simulink model "A2V5"  (R2021b)
settings: Solver=FixedStepAuto  StartTime=0.0  StopTime=10.0  FixedStep=1e-3  RelTol=1e-3  EnableMultiTasking=on
undefined symbols (not defined in the file): a, A0, A1, b, c, D0, D1, D10, D11, D12, D13, D2, D3, D4, D5, D6, D7, D8, D9, magnitude, PTA0, PTA1, PTA2, PTB2, PTB23, PTB3, PTB9, PTC16, PTC17, PTC2, PTC3, PTC4, PTD0, PTD1, PTD2, PTD3
libraries: frdmk64flib x23, etargetslib x21, simulink x2, dspstat3 x1, hdlsllib x1
settings Model: ExtModeTrigDuration=5  Creator=adamj  LastModifiedBy=adamj
settings OptimizationCC: EnhancedBackFolding=on  PassReuseOutputArgsAs=Individual arguments  ZeroExternalMemoryAtStartup=off  ZeroInternalMemoryAtStartup=off  MaxStackSize=64  OptimizeBlockOrder=speed  DifferentSizesBufferReuse=on  OptimizationCustomize=off  EfficientTunableParamExpr=on
settings DebuggingCC: ParameterTunabilityLossMsg=error
settings HardwareCC: ProdBitPerPointer=32  ProdBitPerSizeT=32  ProdBitPerPtrDiffT=32  ProdLargestAtomicInteger=Long  ProdLargestAtomicFloat=Double  ProdWordSize=32  ProdHWDeviceType=ARM Compatible->ARM Cortex
settings SFSimCC: MATLABDynamicMemAlloc=off
settings RTWCC: Description=Embedded Coder  SystemTargetFile=ert.tlc  HardwareBoard=NXP FRDM-K64F  TLCOptions="-aInlineSetEventsForThisBaseRateFcn=TLC_FALSE -aSuppressMultiTaskScheduler=TLC_FALSE  -aRateBasedStepFcn=0"  TemplateMakefile=ert_default_tmf  Toolchain=GNU Tools for ARM Embedded Processors
settings CodeAppCC: ForceParamTrailComments=on  IgnoreCustomStorageClasses=off  OperatorAnnotations=on  SimulinkDataObjDesc=on  SFDataObjDesc=on  InsertBlockDesc=on
settings ERTTargetCC: ExtModeTransport=4  ExtModeMexFile=sendToCommService

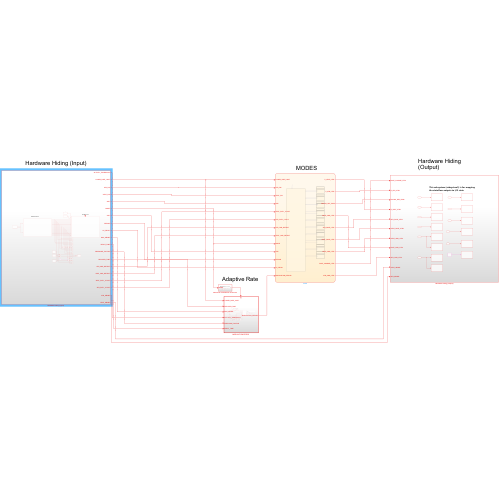
[thumbnail: Simulink's stored preview of the top-level diagram]
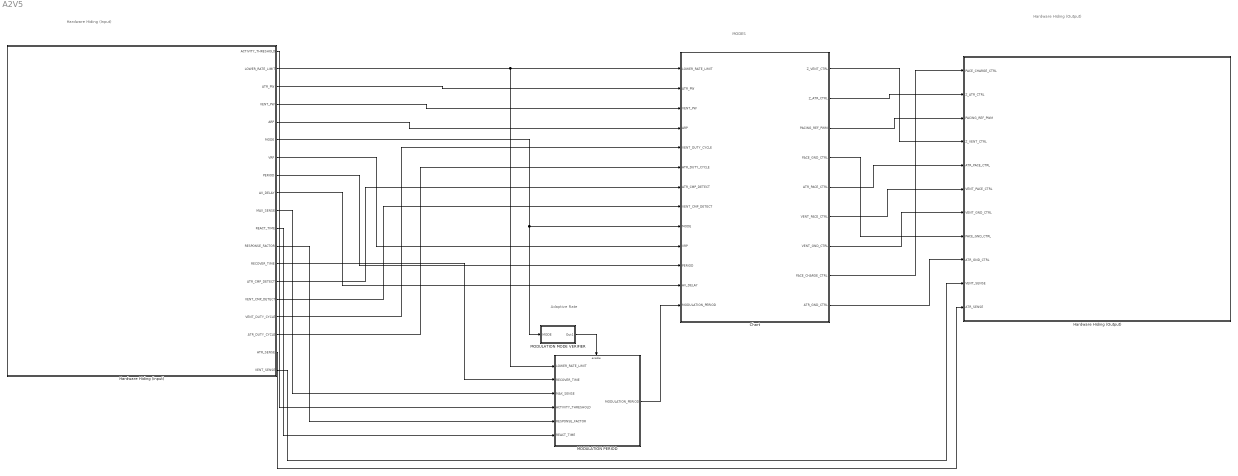
== system A2V5 ==
  note: Hardware Hiding (Output)
  note: Adaptive Rate
  note: MODES
  note: Hardware Hiding (Input)
  Chart : Stateflow chart  TreatAsAtomicUnit=on
  Hardware Hiding (Output) : Subsystem
  Hardware Hiding (input) : Subsystem
  MODULATION MODE VERIFIER : Subsystem
  MODULATION PERIOD : Subsystem
  wires:
  Chart/9(ATR_GND_CTRL) -> Hardware Hiding (Output)/9(ATR_GND_CTRL)
  Chart/2(Z_ATR_CTRL) -> Hardware Hiding (Output)/2(Z_ATR_CTRL)
  Chart/7(VENT_GND_CTRL) -> Hardware Hiding (Output)/7(VENT_GND_CTRL)
  Chart/4(PACE_GND_CTRL) -> Hardware Hiding (Output)/8(PACE_GND_CTRL)
  Chart/8(PACE_CHARGE_CTRL) -> Hardware Hiding (Output)/1(PACE_CHARGE_CTRL)
  Chart/3(PACING_REF_PWM) -> Hardware Hiding (Output)/3(PACING_REF_PWM)
  Chart/5(ATR_PACE_CTRL) -> Hardware Hiding (Output)/5(ATR_PACE_CTRL)
  Chart/1(Z_VENT_CTRL) -> Hardware Hiding (Output)/4(Z_VENT_CTRL)
  Chart/6(VENT_PACE_CTRL) -> Hardware Hiding (Output)/6(VENT_PACE_CTRL)
  MODULATION PERIOD/1(MODULATION_PERIOD) -> Chart/13(MODULATION_PERIOD)
  MODULATION MODE VERIFIER/1(Out1) -> MODULATION PERIOD/Enable
  Hardware Hiding (input)/6(MODE) -> MODULATION MODE VERIFIER/1(MODE), Chart/9(MODE)
  Hardware Hiding (input)/2(LOWER_RATE_LIMIT) -> MODULATION PERIOD/1(LOWER_RATE_LIMIT), Chart/1(LOWER_RATE_LIMIT)
  Hardware Hiding (input)/3(ATR_PW) -> Chart/2(ATR_PW)
  Hardware Hiding (input)/4(VENT_PW) -> Chart/3(VENT_PW)
  Hardware Hiding (input)/5(ARP) -> Chart/4(ARP)
  Hardware Hiding (input)/7(VRP) -> Chart/10(VRP)
  Hardware Hiding (input)/8(PERIOD) -> Chart/11(PERIOD)
  Hardware Hiding (input)/9(AV_DELAY) -> Chart/12(AV_DELAY)
  Hardware Hiding (input)/10(MAX_SENSE) -> MODULATION PERIOD/3(MAX_SENSE)
  Hardware Hiding (input)/11(REACT_TIME) -> MODULATION PERIOD/6(REACT_TIME)
  Hardware Hiding (input)/12(RESPONSE_FACTOR) -> MODULATION PERIOD/5(RESPONSE_FACTOR)
  Hardware Hiding (input)/13(RECOVER_TIME) -> MODULATION PERIOD/2(RECOVER_TIME)
  Hardware Hiding (input)/14(ATR_CMP_DETECT) -> Chart/7(ATR_CMP_DETECT)
  Hardware Hiding (input)/15(VENT_CMP_DETECT) -> Chart/8(VENT_CMP_DETECT)
  Hardware Hiding (input)/16(VENT_DUTY_CYCLE) -> Chart/5(VENT_DUTY_CYCLE)
  Hardware Hiding (input)/17(ATR_DUTY_CYCLE) -> Chart/6(ATR_DUTY_CYCLE)
  Hardware Hiding (input)/1(ACTIVITY_THRESHOLD) -> MODULATION PERIOD/4(ACTIVITY_THRESHOLD)
  Hardware Hiding (input)/19(VENT_SENSE) -> Hardware Hiding (Output)/10(VENT_SENSE)
  Hardware Hiding (input)/18(ATR_SENSE) -> Hardware Hiding (Output)/11(ATR_SENSE)

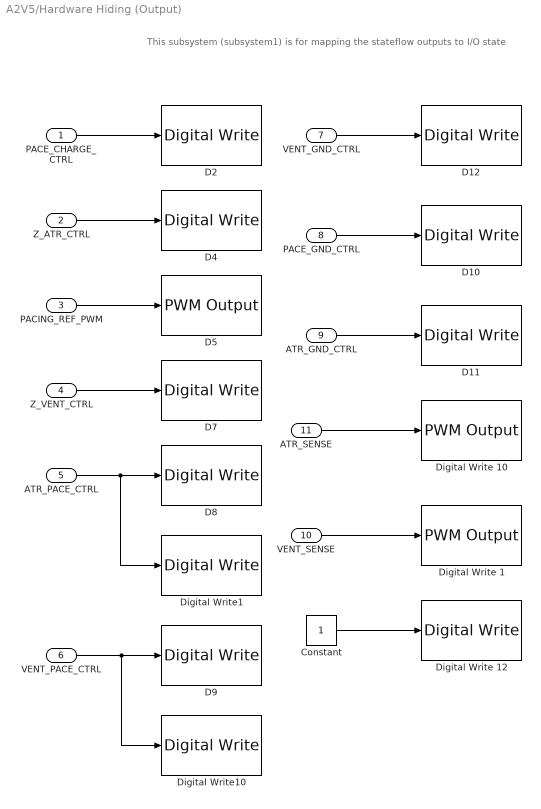
== system A2V5/Hardware Hiding (Output) ==
  note: This subsystem (subsystem1) is for mapping the stateflow outputs to I/O state
  PACE_CHARGE_CTRL : Inport  OutDataTypeStr=boolean
  Z_ATR_CTRL : Inport  Port=2  OutDataTypeStr=boolean
  PACING_REF_PWM : Inport  Port=3  OutDataTypeStr=double
  Z_VENT_CTRL : Inport  Port=4  OutDataTypeStr=boolean
  ATR_PACE_CTRL : Inport  Port=5  OutDataTypeStr=boolean
  VENT_PACE_CTRL : Inport  Port=6  OutDataTypeStr=boolean
  VENT_GND_CTRL : Inport  Port=7  OutDataTypeStr=boolean
  PACE_GND_CTRL : Inport  Port=8  OutDataTypeStr=boolean
  ATR_GND_CTRL : Inport  Port=9  OutDataTypeStr=boolean
  VENT_SENSE : Inport  Port=10
  ATR_SENSE : Inport  Port=11
  Constant : Constant
  D10 : frdmk64flib/Digital Write  Whichpin=PTD0 (D10)
  D11 : frdmk64flib/Digital Write  Whichpin=PTD2 (D11)
  D12 : frdmk64flib/Digital Write  Whichpin=PTD3 (D12)
  D2 : frdmk64flib/Digital Write  Whichpin=PTB9 (D2)
  D4 : frdmk64flib/Digital Write  Whichpin=PTB23 (D4)
  D5 : frdmk64flib/PWM Output  Whichpin=PTA2 (D5)  InitialFrequency=2000  InitialDutyCycle=100
  D7 : frdmk64flib/Digital Write  Whichpin=PTC3 (D7)
  "D8 " : frdmk64flib/Digital Write  Whichpin=PTA0 (D8)
  D9 : frdmk64flib/Digital Write  Whichpin=PTC4 (D9)
  Digital Write 1 : frdmk64flib/PWM Output  Whichpin=PTA1 (D3)  InitialFrequency=2000  InitialDutyCycle=30
  Digital Write 10 : frdmk64flib/PWM Output  Whichpin=PTC2 (D6)  InitialFrequency=2000  InitialDutyCycle=30
  Digital Write 12 : frdmk64flib/Digital Write  Whichpin=PTD1 (D13)
  Digital Write1 : frdmk64flib/Digital Write  Whichpin=BLUE_LED
  Digital Write10 : frdmk64flib/Digital Write  Whichpin=RED_LED
  wires:
  Z_VENT_CTRL/1 -> D7/1
  Z_ATR_CTRL/1 -> D4/1
  PACING_REF_PWM/1 -> D5/1
  VENT_GND_CTRL/1 -> D12/1
  VENT_PACE_CTRL/1 -> Digital Write10/1, D9/1
  ATR_PACE_CTRL/1 -> Digital Write1/1, "D8 "/1
  PACE_CHARGE_CTRL/1 -> D2/1
  PACE_GND_CTRL/1 -> D10/1
  ATR_GND_CTRL/1 -> D11/1
  Constant/1 -> Digital Write 12/1
  VENT_SENSE/1 -> Digital Write 1/1
  ATR_SENSE/1 -> Digital Write 10/1

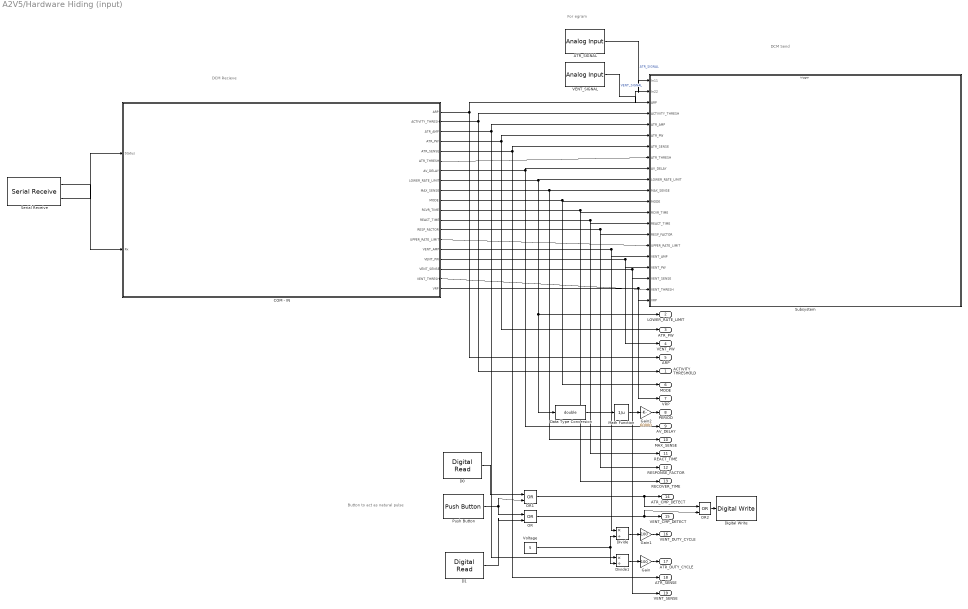
== system A2V5/Hardware Hiding (input) ==
  note: Button to act as natural pulse
  note: For egram
  note: DCM Send
  note: DCM Recieve
  ATR_SIGNAL : frdmk64flib/Analog Input  Whichpin=PTB2 (A0)  SampleTime=-1
  COM - IN : Stateflow chart  TreatAsAtomicUnit=on
  D0 : frdmk64flib/Digital Read  Whichpin=PTC16 (D0)  SampleTime=-1
  D1 : frdmk64flib/Digital Read  Whichpin=PTC17 (D1)  SampleTime=-1
  Data Type Conversion : DataTypeConversion  OutDataTypeStr=double
  Digital Write : frdmk64flib/Digital Write  Whichpin=GREEN_LED
  Divide : Product  Inputs=*/
  Divide1 : Product  Inputs=*/
  Gain : Gain  Gain=100
  Gain1 : Gain  Gain=100
  Gain2 : Gain  Gain=60000  OutDataTypeStr=double
  Math Function : Math  Operator=reciprocal  SaturateOnIntegerOverflow=on
  OR : Logic  Operator=OR  IconShape=distinctive  AllPortsSameDT=off  OutDataTypeStr=boolean
  OR1 : Logic  Operator=OR  IconShape=distinctive  AllPortsSameDT=off  OutDataTypeStr=boolean
  OR2 : Logic  Operator=OR  IconShape=distinctive  AllPortsSameDT=off  OutDataTypeStr=boolean
  Push Button : frdmk64flib/Push Button  Whichswitch=SW3  SampleTime1=-1
  Serial Receive : frdmk64flib/Serial Receive  SCIModule=0  Baudrate=uint32(9600)  Parity=None  StopBits=1  HardwareFlowControl=None  ByteOrder=LittleEndian  DataType=uint8  DataLength=84  BlockingMode=off  OutputStatus=on  SampleTime=-1
  Subsystem : Subsystem
  VENT_SIGNAL : frdmk64flib/Analog Input  Whichpin=PTB3 (A1)  SampleTime=-1
  Voltage : Constant  Value=5
  ACTIVITY_THRESHOLD : Outport
  LOWER_RATE_LIMIT : Outport  Port=2
  ATR_PW : Outport  Port=3
  VENT_PW : Outport  Port=4
  ARP : Outport  Port=5
  MODE : Outport  Port=6
  VRP : Outport  Port=7
  PERIOD : Outport  Port=8
  AV_DELAY : Outport  Port=9
  MAX_SENSE : Outport  Port=10
  REACT_TIME : Outport  Port=11
  RESPONSE_FACTOR : Outport  Port=12
  RECOVER_TIME : Outport  Port=13
  ATR_CMP_DETECT : Outport  Port=14  OutDataTypeStr=boolean
  VENT_CMP_DETECT : Outport  Port=15  OutDataTypeStr=boolean
  VENT_DUTY_CYCLE : Outport  Port=16
  ATR_DUTY_CYCLE : Outport  Port=17
  ATR_SENSE : Outport  Port=18
  VENT_SENSE : Outport  Port=19
  wires:
  COM - IN/7(AV_DELAY) -> AV_DELAY/1, Subsystem/9(AV_DELAY)
  COM - IN/11(RCVR_TIME) -> RECOVER_TIME/1, Subsystem/13(RCVR_TIME)
  COM - IN/13(RESP_FACTOR) -> RESPONSE_FACTOR/1, Subsystem/15(RESP_FACTOR)
  Voltage/1 -> Divide1/2, Divide/2
  Gain/1 -> ATR_DUTY_CYCLE/1
  Divide/1 -> Gain1/1
  COM - IN/2(ACTIVITY_THRESH) -> ACTIVITY_THRESHOLD/1, Subsystem/4(ACTIVITY_THRESH)
  COM - IN/15(VENT_AMP) -> Divide/1, Subsystem/17(VENT_AMP)
  COM - IN/19(VRP) -> VRP/1, Subsystem/21(VRP)
  COM - IN/8(LOWER_RATE_LIMIT) -> Subsystem/10(LOWER_RATE_LIMIT), LOWER_RATE_LIMIT/1, Data Type Conversion/1
  COM - IN/9(MAX_SENSE) -> Subsystem/11(MAX_SENSE), MAX_SENSE/1
  ATR_SIGNAL/1 -> Subsystem/1(In11)  "ATR_SIGNAL"
  COM - IN/17(VENT_SENSE) -> VENT_SENSE/1, Subsystem/19(VENT_SENSE)
  COM - IN/10(MODE) -> Subsystem/12(MODE), MODE/1
  COM - IN/14(UPPER_RATE_LIMIT) -> Subsystem/16(UPPER_RATE_LIMIT)
  COM - IN/6(ATR_THRESH) -> Subsystem/8(ATR_THRESH)
  VENT_SIGNAL/1 -> Subsystem/2(In22)  "VENT_SIGNAL"
  COM - IN/12(REACT_TIME) -> REACT_TIME/1, Subsystem/14(REACT_TIME)
  COM - IN/3(ATR_AMP) -> Divide1/1, Subsystem/5(ATR_AMP)
  Gain1/1 -> VENT_DUTY_CYCLE/1
  COM - IN/16(VENT_PW) -> VENT_PW/1, Subsystem/18(VENT_PW)
  COM - IN/18(VENT_THRESH) -> Subsystem/20(VENT_THRESH)
  COM - IN/5(ATR_SENSE) -> ATR_SENSE/1, Subsystem/7(ATR_SENSE)
  COM - IN/1(ARP) -> ARP/1, Subsystem/3(ARP)
  OR1/1 -> OR2/1, ATR_CMP_DETECT/1
  Divide1/1 -> Gain/1
  COM - IN/4(ATR_PW) -> ATR_PW/1, Subsystem/6(ATR_PW)
  OR2/1 -> Digital Write/1
  OR/1 -> OR2/2, VENT_CMP_DETECT/1
  D1/1 -> OR/2
  Push Button/1 -> OR1/2, OR/1
  Serial Receive/1 -> COM - IN/2(Rx)
  Serial Receive/2 -> COM - IN/1(Status)
  D0/1 -> OR1/1
  Math Function/1 -> Gain2/1
  Gain2/1 -> PERIOD/1
  Data Type Conversion/1 -> Math Function/1

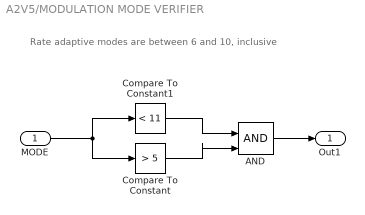
== system A2V5/MODULATION MODE VERIFIER ==
  note: Rate adaptive modes are between 6 and 10, inclusive
  MODE : Inport
  AND : Logic  IconShape=distinctive  AllPortsSameDT=off  OutDataTypeStr=boolean
  Compare To Constant : simulink/Logic and Bit Operations/Compare To Constant  relop=>  const=5  OutDataTypeStr=boolean
  Compare To Constant1 : simulink/Logic and Bit Operations/Compare To Constant  relop=<  const=11  OutDataTypeStr=boolean
  Out1 : Outport
  wires:
  Compare To Constant/1 -> AND/2
  MODE/1 -> Compare To Constant1/1, Compare To Constant/1
  AND/1 -> Out1/1
  Compare To Constant1/1 -> AND/1

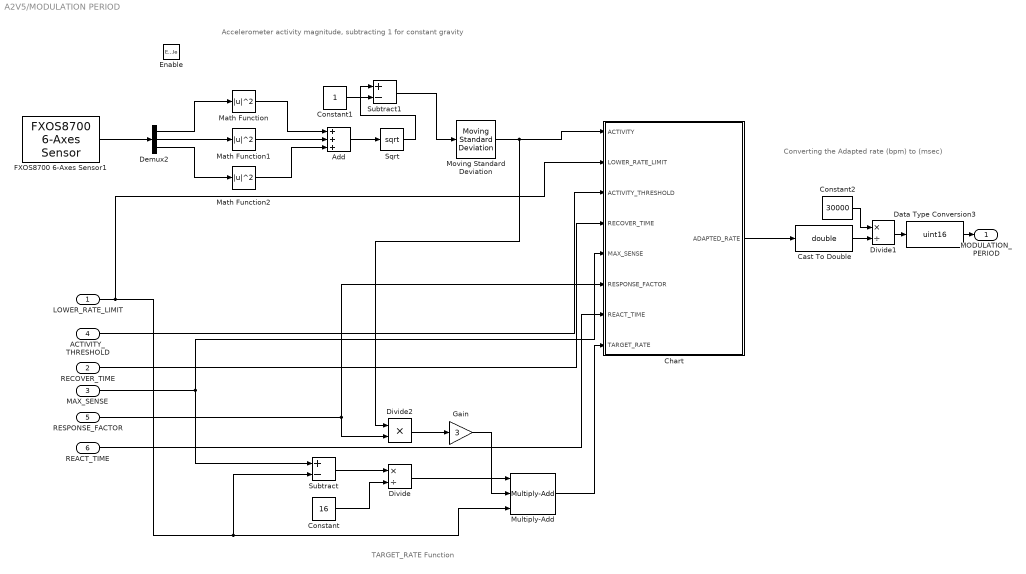
== system A2V5/MODULATION PERIOD ==
  note: Converting the Adapted rate (bpm) to (msec)
  note: Accelerometer activity magnitude, subtracting 1 for constant gravity
  note: TARGET_RATE Function
  LOWER_RATE_LIMIT : Inport
  RECOVER_TIME : Inport  Port=2
  MAX_SENSE : Inport  Port=3
  ACTIVITY_THRESHOLD : Inport  Port=4
  RESPONSE_FACTOR : Inport  Port=5
  REACT_TIME : Inport  Port=6
  Enable : EnablePort
  Add : Sum  Inputs=+++
  Cast To Double : DataTypeConversion  OutDataTypeStr=double
  Chart : Stateflow chart  TreatAsAtomicUnit=on
  Constant : Constant  Value=16
  Constant1 : Constant
  Constant2 : Constant  Value=30000
  Data Type Conversion3 : DataTypeConversion  OutDataTypeStr=uint16
  Demux2 : Demux  Outputs=3
  Divide : Product  Inputs=*/
  Divide1 : Product  Inputs=*/
  Divide2 : Product  Inputs=**  OutDataTypeStr=uint16
  FXOS8700 6-Axes Sensor1 : frdmk64flib/FXOS8700 6-Axes Sensor  Activesensor=Accelerometer only  ODR=800Hz  HybridODR=400Hz  Accelfullrange=-4g to +4g  SampleTime=-1
  Gain : Gain  Gain=3
  Math Function : Math  Operator=magnitude^2  SignedPower=on  OutDataTypeStr=double  SaturateOnIntegerOverflow=on
  Math Function1 : Math  Operator=magnitude^2  SignedPower=on  OutDataTypeStr=double  SaturateOnIntegerOverflow=on
  Math Function2 : Math  Operator=magnitude^2  SignedPower=on  OutDataTypeStr=double  SaturateOnIntegerOverflow=on
  Moving Standard Deviation : dspstat3/Moving Standard Deviation  Method=Sliding window  ForgettingFactorPort=off  SpecifyWindowLength=on  WindowLength=128  ForgettingFactor=0.9  SimulateUsing=Code generation
      settings: SourceProductBaseCode=DS
  Multiply-Add : hdlsllib/HDL Operations/Multiply-Add  Function=c+(a.*b)  datatype=uint8  RndMeth=Nearest  DoSatur=off  FMA=off
      settings: SourceProductBaseCode=SL
  Sqrt : Sqrt  SaturateOnIntegerOverflow=on
  Subtract : Sum  Inputs=+-
  Subtract1 : Sum  Inputs=+-
  MODULATION_PERIOD : Outport
  wires:
  Math Function2/1 -> Add/3
  Demux2/2 -> Math Function1/1
  Math Function/1 -> Add/1
  Add/1 -> Sqrt/1
  Math Function1/1 -> Add/2
  Demux2/1 -> Math Function/1
  Demux2/3 -> Math Function2/1
  FXOS8700 6-Axes Sensor1/1 -> Demux2/1
  Sqrt/1 -> Subtract1/1
  Moving Standard Deviation/1 -> Divide2/1, Chart/1(ACTIVITY)
  ACTIVITY_THRESHOLD/1 -> Chart/3(ACTIVITY_THRESHOLD)
  RECOVER_TIME/1 -> Chart/4(RECOVER_TIME)
  REACT_TIME/1 -> Chart/7(REACT_TIME)
  MAX_SENSE/1 -> Subtract/1, Chart/5(MAX_SENSE)
  Multiply-Add/1 -> Chart/8(TARGET_RATE)
  RESPONSE_FACTOR/1 -> Divide2/2, Chart/6(RESPONSE_FACTOR)
  Divide2/1 -> Gain/1
  Constant2/1 -> Divide1/1
  Constant1/1 -> Subtract1/2
  Subtract1/1 -> Moving Standard Deviation/1
  Cast To Double/1 -> Divide1/2
  Divide1/1 -> Data Type Conversion3/1
  Data Type Conversion3/1 -> MODULATION_PERIOD/1
  LOWER_RATE_LIMIT/1 -> Chart/2(LOWER_RATE_LIMIT), Subtract/2, Multiply-Add/3
  Chart/1(ADAPTED_RATE) -> Cast To Double/1
  Constant/1 -> Divide/2
  Subtract/1 -> Divide/1
  Divide/1 -> Multiply-Add/1
  Gain/1 -> Multiply-Add/2

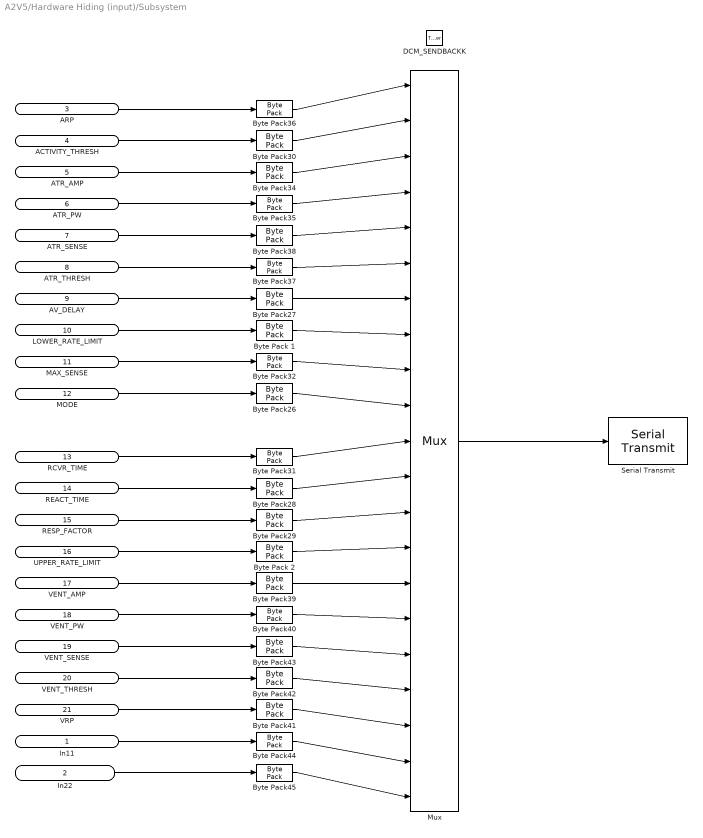
== system A2V5/Hardware Hiding (input)/Subsystem ==
  In11 : Inport
  In22 : Inport  Port=2
  ARP : Inport  Port=3
  ACTIVITY_THRESH : Inport  Port=4
  ATR_AMP : Inport  Port=5
  ATR_PW : Inport  Port=6
  ATR_SENSE : Inport  Port=7
  ATR_THRESH : Inport  Port=8
  AV_DELAY : Inport  Port=9
  LOWER_RATE_LIMIT : Inport  Port=10
  MAX_SENSE : Inport  Port=11
  MODE : Inport  Port=12
  RCVR_TIME : Inport  Port=13
  REACT_TIME : Inport  Port=14
  RESP_FACTOR : Inport  Port=15
  UPPER_RATE_LIMIT : Inport  Port=16
  VENT_AMP : Inport  Port=17
  VENT_PW : Inport  Port=18
  VENT_SENSE : Inport  Port=19
  VENT_THRESH : Inport  Port=20
  VRP : Inport  Port=21
  DCM_SENDBACKK : TriggerPort  TriggerType=function-call  IsSimulinkFunction=on  FunctionName=DCM_SENDBACKK  VariantControl=Variant
  Byte Pack 1 : etargetslib/Byte Pack  datatypes={'uint8'}  byteAlign=1
  Byte Pack 2 : etargetslib/Byte Pack  datatypes={'uint8'}  byteAlign=1
  Byte Pack{26,28..29,31..32,35,40} (7 alike) : etargetslib/Byte Pack  datatypes={'uint8'}  byteAlign=1
  Byte Pack27 : etargetslib/Byte Pack  datatypes={'uint16'}  byteAlign=1
  Byte Pack{30,34,37..39,42..45} (9 alike) : etargetslib/Byte Pack  datatypes={'double'}  byteAlign=1
  Byte Pack36 : etargetslib/Byte Pack  datatypes={'uint16'}  byteAlign=1
  Byte Pack41 : etargetslib/Byte Pack  datatypes={'uint16'}  byteAlign=1
  Mux : Mux  Inputs=21
  Serial Transmit : frdmk64flib/Serial Transmit  SCIModule=0  Baudrate=uint32(9600)  Parity=None  StopBits=1  HardwareFlowControl=None  ByteOrder=LittleEndian  BlockingMode=on  OutputStatus=on
  wires:
  In11/1 -> Byte Pack44/1
  Byte Pack45/1 -> Mux/21
  In22/1 -> Byte Pack45/1
  Byte Pack44/1 -> Mux/20
  Mux/1 -> Serial Transmit/1
  ARP/1 -> Byte Pack36/1
  Byte Pack36/1 -> Mux/1
  Byte Pack30/1 -> Mux/2
  ACTIVITY_THRESH/1 -> Byte Pack30/1
  ATR_AMP/1 -> Byte Pack34/1
  Byte Pack34/1 -> Mux/3
  Byte Pack35/1 -> Mux/4
  ATR_PW/1 -> Byte Pack35/1
  Byte Pack37/1 -> Mux/6
  ATR_THRESH/1 -> Byte Pack37/1
  Byte Pack27/1 -> Mux/7
  AV_DELAY/1 -> Byte Pack27/1
  LOWER_RATE_LIMIT/1 -> Byte Pack 1/1
  Byte Pack 1/1 -> Mux/8
  Byte Pack32/1 -> Mux/9
  MAX_SENSE/1 -> Byte Pack32/1
  MODE/1 -> Byte Pack26/1
  Byte Pack26/1 -> Mux/10
  Byte Pack31/1 -> Mux/11
  RCVR_TIME/1 -> Byte Pack31/1
  Byte Pack28/1 -> Mux/12
  REACT_TIME/1 -> Byte Pack28/1
  Byte Pack29/1 -> Mux/13
  RESP_FACTOR/1 -> Byte Pack29/1
  UPPER_RATE_LIMIT/1 -> Byte Pack 2/1
  Byte Pack 2/1 -> Mux/14
  ATR_SENSE/1 -> Byte Pack38/1
  Byte Pack38/1 -> Mux/5
  Byte Pack40/1 -> Mux/16
  Byte Pack39/1 -> Mux/15
  VENT_AMP/1 -> Byte Pack39/1
  VENT_PW/1 -> Byte Pack40/1
  Byte Pack43/1 -> Mux/17
  VENT_SENSE/1 -> Byte Pack43/1
  VENT_THRESH/1 -> Byte Pack42/1
  Byte Pack42/1 -> Mux/18
  VRP/1 -> Byte Pack41/1
  Byte Pack41/1 -> Mux/19

== stateflow chart A2V5/Chart ==
  state AOO [group]
    state CHARGING
      during:
      %Charge C22 Capacitor
      ATR_PACE_CTRL = LOW
      VENT_PACE_CTRL = LOW
      PACING_REF_PWM = ATR_DUTY_CYCLE
      PACE_CHARGE_CTRL = HIGH
      %Discharge C21 Blocking Capacitor
      PACE_GND_CTRL = HIGH
      VENT_PACE_CTRL = LOW
      Z_ATR_CTRL = LOW
      Z_VENT_CTRL = LOW
      ATR_PACE_CTRL = LOW
      ATR_GND_CTRL = HIGH
      VENT_GND_CTRL = LOW
    state DISCHARGING
      during:
      %Charge C21 Blocking Capacitor
      PACE_CHARGE_CTRL = LOW
      PACE_GND_CTRL = HIGH
      ATR_PACE_CTRL = HIGH %Discharge C22 into Atrium
      ATR_GND_CTRL = LOW
      Z_ATR_CTRL = LOW
      Z_VENT_CTRL = LOW
      VENT_GND_CTRL = LOW
      VENT_PACE_CTRL  = LOW
    AOO.CHARGING -> AOO.DISCHARGING [order 1] : after(PERIOD-ATR_PW, msec)
    AOO.DISCHARGING -> AOO.CHARGING : after(ATR_PW, msec)
  state Start
  state VOO [group]
    state CHARGING
      during:
      %Charge C22 Capacitor
      ATR_PACE_CTRL = LOW
      VENT_PACE_CTRL = LOW
      PACING_REF_PWM = VENT_DUTY_CYCLE
      PACE_CHARGE_CTRL = HIGH
      %Discharge C21 Blocking Capacitor
      PACE_GND_CTRL = HIGH
      VENT_PACE_CTRL = LOW
      Z_ATR_CTRL = LOW
      Z_VENT_CTRL = LOW
      ATR_PACE_CTRL = LOW
      ATR_GND_CTRL = LOW
      VENT_GND_CTRL = HIGH
    state DISCHARGING
      during:
      %Charge Blocking Capacitor
      PACE_CHARGE_CTRL = LOW
      PACE_GND_CTRL = HIGH
      ATR_PACE_CTRL = LOW
      ATR_GND_CTRL = LOW
      Z_ATR_CTRL = LOW
      Z_VENT_CTRL = LOW
      VENT_GND_CTRL = LOW
      VENT_PACE_CTRL  = HIGH %Discharge C22 into Ventricle
    VOO.CHARGING -> VOO.DISCHARGING [order 1] : after(PERIOD-VENT_PW,msec)
    VOO.DISCHARGING -> VOO.CHARGING : after(VENT_PW,msec)
  state AAI [group]
    note: Atrium Sensing For Hysteresis
    state CHARGING
      during:
      %Charge C22 Capacitor
      ATR_PACE_CTRL = LOW
      VENT_PACE_CTRL = LOW
      PACING_REF_PWM = ATR_DUTY_CYCLE
      PACE_CHARGE_CTRL = HIGH
      %Discharge C21 Blocking Capacitor
      PACE_GND_CTRL = HIGH
      VENT_PACE_CTRL = LOW
      Z_ATR_CTRL = LOW
      Z_VENT_CTRL = LOW
      ATR_PACE_CTRL = LOW
      ATR_GND_CTRL = HIGH
      VENT_GND_CTRL = LOW
    state DISCHARGING
      during:
      %Charge Blocking Capacitor
      PACE_CHARGE_CTRL = LOW
      PACE_GND_CTRL = HIGH
      ATR_PACE_CTRL = HIGH %Discharge C22 into Atrium
      ATR_GND_CTRL = LOW
      Z_ATR_CTRL = LOW
      Z_VENT_CTRL = LOW
      VENT_GND_CTRL = LOW
      VENT_PACE_CTRL  = LOW
    note: Atrial Refactory Period
    state CHARGING1
      during:
      %Charge C22 Capacitor
      ATR_PACE_CTRL = LOW
      VENT_PACE_CTRL = LOW
      PACING_REF_PWM = ATR_DUTY_CYCLE
      PACE_CHARGE_CTRL = HIGH
      %Discharge C21 Blocking Capacitor
      PACE_GND_CTRL = HIGH
      VENT_PACE_CTRL = LOW
      Z_ATR_CTRL = LOW
      Z_VENT_CTRL = LOW
      ATR_PACE_CTRL = LOW
      ATR_GND_CTRL = HIGH
      VENT_GND_CTRL = LOW
    (junction 267) -> AAI.CHARGING : after(ARP+uint16(ATR_PW), msec)
    (junction 268) -> (junction 267) [order 1] : [ATR_CMP_DETECT == HIGH]
    (junction 268) -> AAI.DISCHARGING [order 2] : after(uint16(PERIOD)-ARP-uint16(ATR_PW),msec)
    AAI.CHARGING -> (junction 268) [order 1]
    AAI.CHARGING1 -> AAI.CHARGING : after(ARP, msec)
    AAI.DISCHARGING -> AAI.CHARGING1 : after(ATR_PW, msec)
  state VVI [group]
    note: Ventricle Sensing For Hysteresis
    state CHARGING
      during:
      %Charge C22 Capacitor
      ATR_PACE_CTRL = LOW
      VENT_PACE_CTRL = LOW
      PACING_REF_PWM = VENT_DUTY_CYCLE
      PACE_CHARGE_CTRL = HIGH
      %Discharge Blocking Capacitor
      PACE_GND_CTRL = HIGH
      VENT_PACE_CTRL = LOW
      Z_ATR_CTRL = LOW
      Z_VENT_CTRL = LOW
      ATR_PACE_CTRL = LOW
      ATR_GND_CTRL = LOW
      VENT_GND_CTRL = HIGH
    state DISCHARGING
      during:
      %Charge Blocking Capacitor
      PACE_CHARGE_CTRL = LOW
      PACE_GND_CTRL = HIGH
      ATR_PACE_CTRL = LOW
      ATR_GND_CTRL = LOW
      Z_ATR_CTRL = LOW
      Z_VENT_CTRL = LOW
      VENT_GND_CTRL = LOW
      VENT_PACE_CTRL  = HIGH %Discharge C22 into Ventricle
    state CHARGING1
      during:
      %Charge C22 Capacitor
      ATR_PACE_CTRL = LOW
      VENT_PACE_CTRL = LOW
      PACING_REF_PWM = VENT_DUTY_CYCLE
      PACE_CHARGE_CTRL = HIGH
      %Discharge Blocking Capacitor
      PACE_GND_CTRL = HIGH
      VENT_PACE_CTRL = LOW
      Z_ATR_CTRL = LOW
      Z_VENT_CTRL = LOW
      ATR_PACE_CTRL = LOW
      ATR_GND_CTRL = LOW
      VENT_GND_CTRL = HIGH
    note: Ventricular Refractory Period
    (junction 252) -> VVI.CHARGING : after(VENT_PW, msec)
    (junction 248) -> (junction 252) [order 1] : [VENT_CMP_DETECT == HIGH]
    (junction 248) -> VVI.DISCHARGING [order 2] : after(uint16(PERIOD)-VRP-uint16(VENT_PW),msec)
    VVI.CHARGING -> (junction 248) [order 2]
    VVI.CHARGING1 -> VVI.CHARGING : after(VRP, msec)
    VVI.DISCHARGING -> VVI.CHARGING1 : after(VENT_PW, msec)
  state DOO [group]
    state ATR_CHARGING
      during:
      %Begin Charging C22 Capacitor
      ATR_PACE_CTRL = LOW
      VENT_PACE_CTRL = LOW
      PACING_REF_PWM = ATR_DUTY_CYCLE
      PACE_CHARGE_CTRL = HIGH
      %Begin Discharging C21 Blocking Capacitor
      PACE_GND_CTRL = HIGH
      VENT_PACE_CTRL = LOW
      Z_ATR_CTRL = LOW
      Z_VENT_CTRL = LOW
      ATR_PACE_CTRL = LOW
      ATR_GND_CTRL = HIGH
      VENT_GND_CTRL = LOW
    state VENT_CHARGING
      during:
      %Begin Charging C22 Capacitor
      ATR_PACE_CTRL = LOW
      VENT_PACE_CTRL = LOW
      PACING_REF_PWM = VENT_DUTY_CYCLE
      PACE_CHARGE_CTRL = HIGH
      %Begin Discharging C21 Blocking Capacitor
      PACE_GND_CTRL = HIGH
      VENT_PACE_CTRL = LOW
      Z_ATR_CTRL = LOW
      Z_VENT_CTRL = LOW
      ATR_PACE_CTRL = LOW
      ATR_GND_CTRL = LOW
      VENT_GND_CTRL = HIGH
    state ATR_DISCHARGING
      during:
      %Discharge C22 into Atrium
      %Begin Charging C21 Blocking Capacitor
      PACE_CHARGE_CTRL = LOW
      PACE_GND_CTRL = HIGH
      ATR_PACE_CTRL = HIGH
      ATR_GND_CTRL = LOW
      Z_ATR_CTRL = LOW
      Z_VENT_CTRL = LOW
      VENT_GND_CTRL = LOW
      VENT_PACE_CTRL  = LOW
    state VENT_DISCHARGING
      during:
      %Discharge C22 into Ventricle (Vent Pacing)
      %Begin Charging Blocking Capacitor
      PACE_CHARGE_CTRL = LOW
      PACE_GND_CTRL = HIGH
      ATR_PACE_CTRL = LOW
      ATR_GND_CTRL = LOW
      Z_ATR_CTRL = LOW
      Z_VENT_CTRL = LOW
      VENT_GND_CTRL = LOW
      VENT_PACE_CTRL  = HIGH
    VENT_DISCHARGING -> VENT_CHARGING : after(VENT_PW,msec)
    ATR_DISCHARGING -> ATR_CHARGING : after(ATR_PW, msec)
    ATR_CHARGING -> VENT_DISCHARGING : after(AV_DELAY-uint16(ATR_PW),msec)
    VENT_CHARGING -> ATR_DISCHARGING [order 1] : after(uint16(PERIOD) - uint16(VENT_PW) - AV_DELAY, msec)
  state DOOR [group]
    state ATR_CHARGING2
      during:
      %Begin Charging C22 Capacitor
      ATR_PACE_CTRL = LOW
      VENT_PACE_CTRL = LOW
      PACING_REF_PWM = VENT_DUTY_CYCLE
      PACE_CHARGE_CTRL = HIGH
      %Begin Discharging C21 Blocking Capacitor
      PACE_GND_CTRL = HIGH
      VENT_PACE_CTRL = LOW
      Z_ATR_CTRL = LOW
      Z_VENT_CTRL = LOW
      ATR_PACE_CTRL = LOW
      ATR_GND_CTRL = HIGH
      VENT_GND_CTRL = LOW
    state VENT_CHARGING1
      during:
      %Begin Charging C22 Capacitor
      ATR_PACE_CTRL = LOW
      VENT_PACE_CTRL = LOW
      PACING_REF_PWM = ATR_DUTY_CYCLE
      PACE_CHARGE_CTRL = HIGH
      %Begin Discharging C21 Blocking Capacitor
      PACE_GND_CTRL = HIGH
      VENT_PACE_CTRL = LOW
      Z_ATR_CTRL = LOW
      Z_VENT_CTRL = LOW
      ATR_PACE_CTRL = LOW
      ATR_GND_CTRL = LOW
      VENT_GND_CTRL = HIGH
    state ATR_DISCHARGING1
      during:
      %Discharge C22 into Atrium (AtrialPacing)
      %Begin Charging C21 Blocking Capacitor
      PACE_CHARGE_CTRL = LOW
      PACE_GND_CTRL = HIGH
      ATR_PACE_CTRL = HIGH
      ATR_GND_CTRL = LOW
      Z_ATR_CTRL = LOW
      Z_VENT_CTRL = LOW
      VENT_GND_CTRL = LOW
      VENT_PACE_CTRL  = LOW
    state VENT_DISCHARGING1
      during:
      %Discharge C22 into Ventricle (Vent Pacing)
      %Begin Charging Blocking Capacitor
      PACE_CHARGE_CTRL = LOW
      PACE_GND_CTRL = HIGH
      ATR_PACE_CTRL = LOW
      ATR_GND_CTRL = LOW
      Z_ATR_CTRL = LOW
      Z_VENT_CTRL = LOW
      VENT_GND_CTRL = LOW
      VENT_PACE_CTRL  = HIGH
    VENT_DISCHARGING1 -> ATR_CHARGING2 : after(VENT_PW,msec)
    ATR_DISCHARGING1 -> VENT_CHARGING1 : after(ATR_PW, msec)
    VENT_CHARGING1 -> VENT_DISCHARGING1 : after(AV_DELAY-uint16(ATR_PW),msec)
    ATR_CHARGING2 -> ATR_DISCHARGING1 [order 2] : after(MODULATION_PERIOD - uint16(VENT_PW) - AV_DELAY, msec)
  state AOOR [group]
    state CHARGING
      during:
      %Begin Charging C22 Capacitor
      ATR_PACE_CTRL = LOW
      VENT_PACE_CTRL = LOW
      PACING_REF_PWM = ATR_DUTY_CYCLE
      PACE_CHARGE_CTRL = HIGH
      %Begin Discharging C21 Blocking Capacitor
      PACE_GND_CTRL = HIGH
      VENT_PACE_CTRL = LOW
      Z_ATR_CTRL = LOW
      Z_VENT_CTRL = LOW
      ATR_PACE_CTRL = LOW
      ATR_GND_CTRL = HIGH
      VENT_GND_CTRL = LOW
    state DISCHARGING
      during:
      %Discharge C22 into Atrium (AtrialPacing)
      %Begin Charging C21 Blocking Capacitor
      PACE_CHARGE_CTRL = LOW
      PACE_GND_CTRL = HIGH
      ATR_PACE_CTRL = HIGH
      ATR_GND_CTRL = LOW
      Z_ATR_CTRL = LOW
      Z_VENT_CTRL = LOW
      VENT_GND_CTRL = LOW
      VENT_PACE_CTRL  = LOW
    AOOR.CHARGING -> AOOR.DISCHARGING [order 1] : after(MODULATION_PERIOD - uint16(ATR_PW), msec)
    AOOR.DISCHARGING -> AOOR.CHARGING : after(ATR_PW, msec)
  state VOOR [group]
    state CHARGING
      during:
      %Begin Charging C22 Capacitor
      ATR_PACE_CTRL = LOW
      VENT_PACE_CTRL = LOW
      PACING_REF_PWM = VENT_DUTY_CYCLE
      PACE_CHARGE_CTRL = HIGH
      %Begin Discharging C21 Blocking Capacitor
      PACE_GND_CTRL = HIGH
      VENT_PACE_CTRL = LOW
      Z_ATR_CTRL = LOW
      Z_VENT_CTRL = LOW
      ATR_PACE_CTRL = LOW
      ATR_GND_CTRL = LOW
      VENT_GND_CTRL = HIGH
    state DISCHARGING
      during:
      %Discharge C22 into Ventricle (Vent Pacing)
      %Begin Charging Blocking Capacitor
      PACE_CHARGE_CTRL = LOW
      PACE_GND_CTRL = HIGH
      ATR_PACE_CTRL = LOW
      ATR_GND_CTRL = LOW
      Z_ATR_CTRL = LOW
      Z_VENT_CTRL = LOW
      VENT_GND_CTRL = LOW
      VENT_PACE_CTRL  = HIGH
    VOOR.CHARGING -> VOOR.DISCHARGING [order 1] : after(MODULATION_PERIOD - uint16(VENT_PW), msec)
    VOOR.DISCHARGING -> VOOR.CHARGING : after(VENT_PW,msec)
  state AAIR [group]
    note: Atrium Sensing For Hysteresis
    state CHARGING
      during:
      %Charge C22 Capacitor
      ATR_PACE_CTRL = LOW
      VENT_PACE_CTRL = LOW
      PACING_REF_PWM = ATR_DUTY_CYCLE
      PACE_CHARGE_CTRL = HIGH
      %Discharge C21 Blocking Capacitor
      PACE_GND_CTRL = HIGH
      VENT_PACE_CTRL = LOW
      Z_ATR_CTRL = LOW
      Z_VENT_CTRL = LOW
      ATR_PACE_CTRL = LOW
      ATR_GND_CTRL = HIGH
      VENT_GND_CTRL = LOW
    state DISCHARGING
      during:
      %Charge Blocking Capacitor
      PACE_CHARGE_CTRL = LOW
      PACE_GND_CTRL = HIGH
      ATR_PACE_CTRL = HIGH %Discharge C22 into Atrium
      ATR_GND_CTRL = LOW
      Z_ATR_CTRL = LOW
      Z_VENT_CTRL = LOW
      VENT_GND_CTRL = LOW
      VENT_PACE_CTRL  = LOW
    note: Atrial Refactory Period
    state CHARGING1
      during:
      %Charge C22 Capacitor
      ATR_PACE_CTRL = LOW
      VENT_PACE_CTRL = LOW
      PACING_REF_PWM = ATR_DUTY_CYCLE
      PACE_CHARGE_CTRL = HIGH
      %Discharge C21 Blocking Capacitor
      PACE_GND_CTRL = HIGH
      VENT_PACE_CTRL = LOW
      Z_ATR_CTRL = LOW
      Z_VENT_CTRL = LOW
      ATR_PACE_CTRL = LOW
      ATR_GND_CTRL = HIGH
      VENT_GND_CTRL = LOW
    (junction 390) -> AAIR.CHARGING : after(ATR_PW, msec)
    (junction 396) -> (junction 390) [order 1] : [ATR_CMP_DETECT == HIGH]
    (junction 396) -> AAIR.DISCHARGING [order 2] : after(MODULATION_PERIOD-ARP-uint16(ATR_PW),msec)
    AAIR.CHARGING -> (junction 396) [order 1]
    AAIR.CHARGING1 -> AAIR.CHARGING : after(ARP, msec)
    AAIR.DISCHARGING -> AAIR.CHARGING1 : after(ATR_PW, msec)
  state VVIR [group]
    note: Ventricle Sensing For Hysteresis
    state CHARGING
      during:
      %Charge C22 Capacitor
      ATR_PACE_CTRL = LOW
      VENT_PACE_CTRL = LOW
      PACING_REF_PWM = VENT_DUTY_CYCLE
      PACE_CHARGE_CTRL = HIGH
      %Discharge Blocking Capacitor
      PACE_GND_CTRL = HIGH
      VENT_PACE_CTRL = LOW
      Z_ATR_CTRL = LOW
      Z_VENT_CTRL = LOW
      ATR_PACE_CTRL = LOW
      ATR_GND_CTRL = LOW
      VENT_GND_CTRL = HIGH
    state DISCHARGING
      during:
      %Charge Blocking Capacitor
      PACE_CHARGE_CTRL = LOW
      PACE_GND_CTRL = HIGH
      ATR_PACE_CTRL = LOW
      ATR_GND_CTRL = LOW
      Z_ATR_CTRL = LOW
      Z_VENT_CTRL = LOW
      VENT_GND_CTRL = LOW
      VENT_PACE_CTRL  = HIGH %Discharge C22 into Ventricle
    note: Ventricular Refractory Period
    state CHARGING1
      during:
      %Charge C22 Capacitor
      ATR_PACE_CTRL = LOW
      VENT_PACE_CTRL = LOW
      PACING_REF_PWM = VENT_DUTY_CYCLE
      PACE_CHARGE_CTRL = HIGH
      %Discharge Blocking Capacitor
      PACE_GND_CTRL = HIGH
      VENT_PACE_CTRL = LOW
      Z_ATR_CTRL = LOW
      Z_VENT_CTRL = LOW
      ATR_PACE_CTRL = LOW
      ATR_GND_CTRL = LOW
      VENT_GND_CTRL = HIGH
    (junction 413) -> VVIR.CHARGING : after(VENT_PW, msec)
    (junction 408) -> (junction 413) [order 1] : [VENT_CMP_DETECT == HIGH]
    (junction 408) -> VVIR.DISCHARGING [order 2] : after(MODULATION_PERIOD-VRP-uint16(VENT_PW),msec)
    VVIR.CHARGING -> (junction 408) [order 1]
    VVIR.CHARGING1 -> VVIR.CHARGING : after(VRP, msec)
    VVIR.DISCHARGING -> VVIR.CHARGING1 : after(VENT_PW, msec)
  Start -> VVIR.CHARGING [order 9] : [MODE == 10]
  Start -> ATR_CHARGING2 [order 6] : [MODE == 6]
  Start -> AOOR.CHARGING [order 7] : [MODE == 7]
  Start -> VOOR.CHARGING [order 8] : [MODE == 8]
  Start -> AAIR.CHARGING [order 10] : [MODE == 9]
  ATR_CHARGING2 -> Start [order 1] : [MODE ~= 6]
  VENT_CHARGING -> Start [order 2] : [MODE ~= 5]
  AAI.CHARGING -> Start [order 2] : [MODE ~= 3]
  Start -> AAI.CHARGING [order 3] : [MODE == 3]
  Start -> VOO.CHARGING [order 2] : [MODE == 2]
  AOOR.CHARGING -> Start [order 2] : [MODE ~= 7]
  AAIR.CHARGING -> Start [order 2] : [MODE ~= 9]
  VOO.CHARGING -> Start [order 2] : [MODE ~= 2]
  VOOR.CHARGING -> Start [order 2] : [MODE ~= 8]
  (default) -> Start
  VVIR.CHARGING -> Start [order 2] : [MODE ~= 10]
  Start -> VENT_CHARGING [order 5] : [MODE == 5]
  Start -> VVI.CHARGING [order 4] : [MODE == 4]
  AOO.CHARGING -> Start [order 2] : [MODE ~= 1]
  VVI.CHARGING -> Start [order 1] : [MODE ~= 4]
  Start -> AOO.CHARGING [order 1] : [MODE == 1]
  data: LOWER_RATE_LIMIT input; ATR_PW input; VENT_PW input; ARP input; VENT_DUTY_CYCLE input; ATR_DUTY_CYCLE input; ATR_CMP_DETECT input; VENT_CMP_DETECT input boolean; MODE input; VRP input; PERIOD input; Z_VENT_CTRL output; Z_ATR_CTRL output; PACING_REF_PWM output; PACE_GND_CTRL output boolean; ATR_PACE_CTRL output boolean; VENT_PACE_CTRL output boolean; VENT_GND_CTRL output boolean; PACE_CHARGE_CTRL output boolean; ATR_GND_CTRL output; HIGH local boolean =true; LOW local =false; AV_DELAY input; MODULATION_PERIOD input

== stateflow chart A2V5/MODULATION PERIOD/Chart ==
  state State1
    entry:
    step_up = uint8(ceil((MAX_SENSE - LOWER_RATE_LIMIT) / REACT_TIME))
    step_down = uint8(ceil((MAX_SENSE - LOWER_RATE_LIMIT)  / RECOVER_TIME))
    ADAPTED_RATE = LOWER_RATE_LIMIT;
  state IncreasedRate
    entry:
    ADAPTED_RATE = ADAPTED_RATE + step_up;
  state State3
    entry:
    ADAPTED_RATE = TARGET_RATE;
  state BUFFER
    entry:
    ADAPTED_RATE = ADAPTED_RATE - step_up;
  state DecreasedRate
    entry:
    ADAPTED_RATE = ADAPTED_RATE - step_down;
  (default) -> State1
  IncreasedRate -> IncreasedRate [order 1] : after(1000,msec)[ADAPTED_RATE <= MAX_SENSE]
  State3 -> State3 [order 2] : [ACTIVITY > ACTIVITY_THRESHOLD]
  IncreasedRate -> State3 [order 3] : [ADAPTED_RATE >= MAX_SENSE]
  State1 -> State1 [order 2] : [ACTIVITY < ACTIVITY_THRESHOLD]
  State1 -> IncreasedRate [order 1] : [ACTIVITY >= ACTIVITY_THRESHOLD]
  IncreasedRate -> BUFFER [order 2] : [ACTIVITY <  ACTIVITY_THRESHOLD]
  BUFFER -> IncreasedRate [order 1] : [ACTIVITY >= ACTIVITY_THRESHOLD]
  DecreasedRate -> IncreasedRate [order 3] : [ACTIVITY >= ACTIVITY_THRESHOLD]
  DecreasedRate -> State1 [order 1] : [ADAPTED_RATE <= LOWER_RATE_LIMIT]
  State3 -> DecreasedRate [order 1] : [ACTIVITY < ACTIVITY_THRESHOLD]
  BUFFER -> DecreasedRate [order 2] : [ after(1000,msec)]
  DecreasedRate -> DecreasedRate [order 2] : after(1000, msec)[ADAPTED_RATE >= LOWER_RATE_LIMIT]
  data: ACTIVITY input; step_up local uint8; step_down local uint8; LOWER_RATE_LIMIT input uint8; ACTIVITY_THRESHOLD input; RECOVER_TIME input; MAX_SENSE input; RESPONSE_FACTOR input; REACT_TIME input; TARGET_RATE input; ADAPTED_RATE output uint8

== stateflow chart A2V5/Hardware Hiding (input)/COM - IN ==
  note: ?
  state Default
    %Setting values to variables if
    %not initialized in DCM
    entry:
    %GENERAL
    MODE = 10;
    LOWER_RATE_LIMIT = 60;
    UPPER_RATE_LIMIT = 120;
    AV_DELAY = 150;
    REACT_TIME = 10;
    RESP_FACTOR = 16;
    ACTIVITY_THRESH = 1;
    RCVR_TIME = 20;
    MAX_SENSE = 180;
    %ATRIUM
    ATR_AMP = 3.5;
    ATR_PW = 10;
    ARP = 200;
    ATR_THRESH = 1.8;
    ATR_SENSE = 70;
    %VENTRICLE
    VENT_AMP = 3.5;
    VENT_PW = 10;
    VRP = 200;
    VENT_THRESH = 2.2;
    VENT_SENSE = 70;
  state SET_PARAM
    entry:
    MODE = typecast(Rx(3), 'uint8');
    LOWER_RATE_LIMIT = typecast(Rx(4), 'uint8');
    UPPER_RATE_LIMIT = typecast(Rx(5), 'uint8');
    AV_DELAY = typecast(Rx(6:7), 'uint16');
    REACT_TIME = typecast(Rx(8), 'uint8');
    RESP_FACTOR = typecast(Rx(9), 'uint8');
    ACTIVITY_THRESH = typecast(Rx(10:17), 'double');
    RCVR_TIME = typecast(Rx(18), 'uint8');
    MAX_SENSE = typecast(Rx(19), 'uint8');
    %ATR
    ATR_AMP = typecast(Rx(20:27), 'double');
    ATR_PW = typecast(Rx(28), 'uint8');
    ARP = typecast(Rx(29:30), 'uint16');
    ATR_THRESH = typecast(Rx(31:38), 'double');
    ATR_SENSE = typecast(Rx(39:46), 'double');
    %VENT
    VENT_AMP = typecast(Rx(47:54), 'double');
    VENT_PW = typecast(Rx(55), 'uint8');
    VRP = typecast(Rx(56:57), 'uint16');
    VENT_THRESH = typecast(Rx(58:65), 'double');
    VENT_SENSE = typecast(Rx(66:73), 'double');
  state STANDBY
  state ECHO_PARAM
    entry:
    DCM_SENDING();
  (default) -> Default
  SET_PARAM -> STANDBY
  (junction 31) -> STANDBY [order 2]
  Default -> STANDBY
  STANDBY -> (junction 31) : [Status == 0]
  (junction 31) -> (junction 37) [order 1] : [Rx(1) == hex2dec('16')]
  (junction 37) -> SET_PARAM [order 2] : [Rx(2) == hex2dec('55')]
  (junction 37) -> ECHO_PARAM [order 1] : [Rx(2) == hex2dec('22')]
  ECHO_PARAM -> STANDBY
  data: Status input uint8; Rx input uint8; ARP output uint16; ACTIVITY_THRESH output double; ATR_AMP output double; ATR_PW output uint8; ATR_SENSE output double; ATR_THRESH output double; AV_DELAY output uint16; LOWER_RATE_LIMIT output uint8; MAX_SENSE output uint8; MODE output uint8; RCVR_TIME output uint8; REACT_TIME output uint8; RESP_FACTOR output uint8; UPPER_RATE_LIMIT output uint8; VENT_AMP output double; VENT_PW output uint8; VENT_SENSE output double; VENT_THRESH output double; VRP output uint16
